simulink model "nmpc"  (R2024b)
settings: Solver=ode4  StartTime=0.0  StopTime=15  FixedStep=0.02  RelTol=1e-3
libraries: mpclib x1
settings Model: Creator=Manuela  LastModifiedBy=Manuela

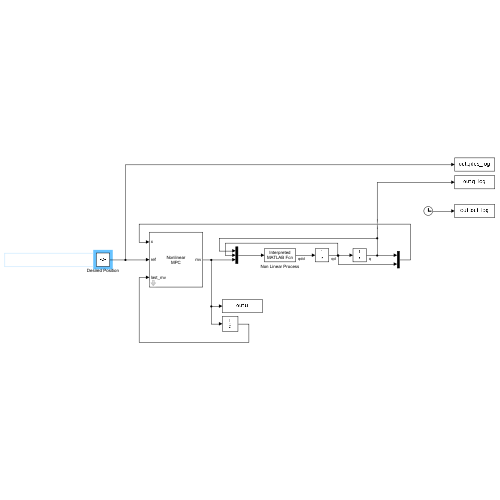
[thumbnail: Simulink's stored preview of the top-level diagram]
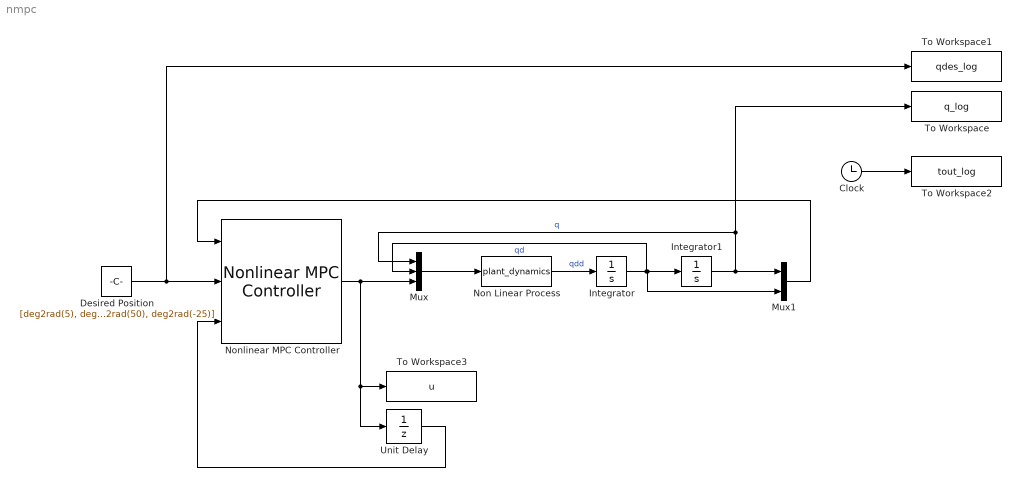
== system nmpc ==
  Clock : Clock
  Desired Position : Constant  Value=[deg2rad(5), deg2rad(50), deg2rad(-25)]  VectorParams1D=off  SampleTime=0.2
  Integrator : Integrator  InitialCondition=zeros(3,1)
  Integrator1 : Integrator  InitialCondition=[0; pi/4; -pi/6]
  Mux : Mux  Inputs=3
  Mux1 : Mux  Inputs=2
  Non Linear Process : MATLABFcn  MATLABFcn=plant_dynamics  OutputDimensions=3
  Nonlinear MPC Controller : mpclib/Nonlinear MPC Controller  nlmpcobj=nlobj  UseObjectTs=on  UseMEX=off  md_enabled=off  mvtarget_enabled=off  param_enabled=off  cost_enabled=off  mvseq_enabled=off  stateseq_enabled=off  ovseq_enabled=off  slack_enabled=off  status_enabled=off  ov_min=off  ov_max=off  mv_min=off  mv_max=off  mvrate_min=off  mvrate_max=off  state_min=off  state_max=off  ov_weight=off  mv_weight=off  mvrate_weight=off  ecr_weight=off  nlp_initialize=off
  To Workspace : ToWorkspace  VariableName=q_log  SampleTime=-1
  To Workspace1 : ToWorkspace  VariableName=qdes_log  SampleTime=0.02
  To Workspace2 : ToWorkspace  VariableName=tout_log  SampleTime=-1
  To Workspace3 : ToWorkspace  VariableName=u  SampleTime=0.02
  Unit Delay : UnitDelay  SampleTime=-1  HasFrameUpgradeWarning=on
  wires:
  Clock/1 -> To Workspace2/1
  Desired Position/1 -> To Workspace1/1, Nonlinear MPC Controller/2
  Nonlinear MPC Controller/1 -> Unit Delay/1, To Workspace3/1, Mux/3
  Mux/1 -> Non Linear Process/1
  Non Linear Process/1 -> Integrator/1  "qdd"
  Integrator/1 -> Mux/2, Mux1/2, Integrator1/1  "qd"
  Integrator1/1 -> To Workspace/1, Mux/1, Mux1/1  "q"
  Mux1/1 -> Nonlinear MPC Controller/1
  Unit Delay/1 -> Nonlinear MPC Controller/3
